simulink model "AW_1"  (R2016b)
settings: Solver=VariableStepAuto  StartTime=0.0  StopTime=15  RelTol=1e-3
values from neighbouring files (symbols this model uses):
  CC = ss(C)    [H_inf_syn_3_mass.m]    (also in prova_con_state_feedback.m = ss( zeros(2),zeros(2) , zeros(2) , [K(1) 0; 0 K(2)] ))
  GG = ss(G)    [H_inf_syn_3_mass.m]    (also in prova_con_state_feedback.m = ss([0 -3;0 -4],2*ones(2,1),eye(2),zeros(2,1)))
settings Model: Creator=giamm  LastModifiedBy=giamm

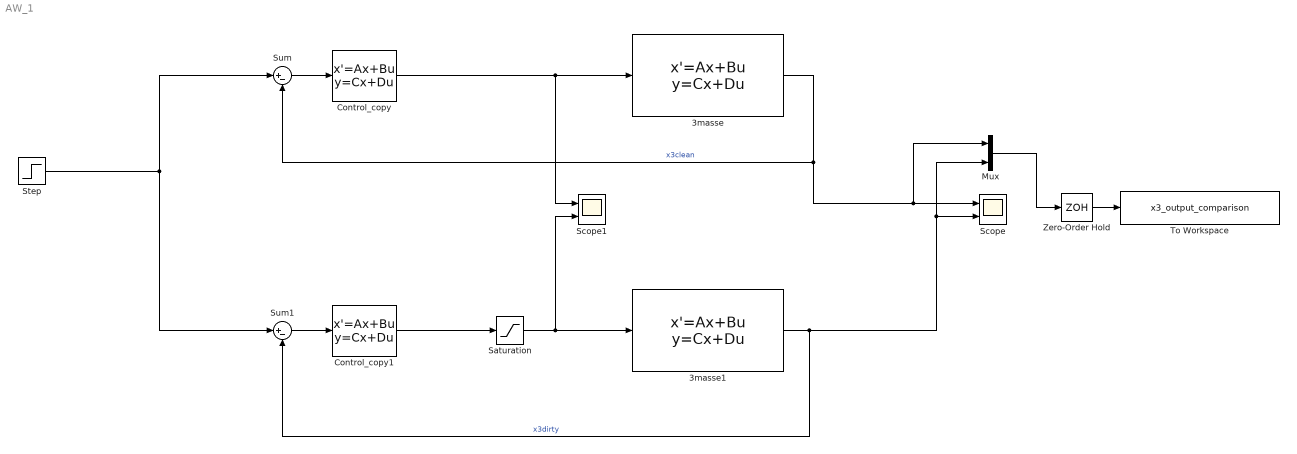
== system AW_1 ==
  3masse : StateSpace  A=GG.A  B=GG.B  C=GG.C  D=GG.D  X0=[0 0 0 0 0 0]
  3masse1 : StateSpace  A=GG.A  B=GG.B  C=GG.C  D=GG.D  X0=[0 0 0 0 0 0]
  Control_copy : StateSpace  A=CC.A  B=CC.B  C=CC.C  D=CC.D  X0=[0 0 0]
  Control_copy1 : StateSpace  A=CC.A  B=CC.B  C=CC.C  D=CC.D  X0=[0 0 0]
  Mux : Mux  Inputs=2
  Saturation : Saturate  UpperLimit=0.1  LowerLimit=-0.1
  Scope : Scope  NumInputPorts=2
  Scope1 : Scope  NumInputPorts=2
  Step : Step  After=0.02  SampleTime=0
  Sum : Sum  Inputs=|+-
  Sum1 : Sum  Inputs=|+-
  To Workspace : ToWorkspace  VariableName=x3_output_comparison  SaveFormat=Structure With Time  SampleTime=-1
  Zero-Order Hold : ZeroOrderHold  SampleTime=0.005
  wires:
  3masse/1 -> Sum/2, Mux/1, Scope/1  "x3clean"
  3masse1/1 -> Sum1/2, Mux/2, Scope/2  "x3dirty"
  Sum/1 -> Control_copy/1
  Step/1 -> Sum/1, Sum1/1
  Control_copy1/1 -> Saturation/1
  Sum1/1 -> Control_copy1/1
  Control_copy/1 -> 3masse/1, Scope1/1
  Saturation/1 -> 3masse1/1, Scope1/2
  Mux/1 -> Zero-Order Hold/1
  Zero-Order Hold/1 -> To Workspace/1
